simulink model "Allapotvisszacsatolas"  (Simulink 8.7)
settings: Solver=VariableStepAuto  StartTime=0.0  StopTime=T_sim  FixedStep=0.001  RelTol=1e-3
values from neighbouring files (symbols this model uses):
  d = 0.065    [Allapotvisszacsatolas_sim.m]
  delta_0 = deg2rad(delta_0)    [Allapotvisszacsatolas_sim.m]
  fi_0 = pi*fi_0*(SERVO_BAL-SERVO_JOBB)/(360*fi_m)    (= 0)    [Allapotvisszacsatolas_sim.m]
  fi_m = deg2rad(fi_m)    [Allapotvisszacsatolas_sim.m]
  k_delta = (L+d)/(kszi^2*d_5s^2)*(9*(L+d)-6*kszi^2*d_5s)    (= -0.808096379979)    [Allapotvisszacsatolas_sim.m]
  k_p = -9*(L+d)/(kszi^2*d_5s^2)    (= -3.12434564743)    [Allapotvisszacsatolas_sim.m]
  L = 0.22    [Allapotvisszacsatolas_sim.m]
  L_sensor = 0.13    [Allapotvisszacsatolas_sim.m]
  m = deg2rad(m)    [Allapotvisszacsatolas_sim.m]
  p_0 = 0.06    [Allapotvisszacsatolas_sim.m]
  p_1s = 0.0917605    [Allapotvisszacsatolas_sim.m]
  p_1TCRTa = 100    [Allapotvisszacsatolas_sim.m]
  p_1TCRTb = 3200    [Allapotvisszacsatolas_sim.m]
  p_2s = 0.068075    [Allapotvisszacsatolas_sim.m]
  p_2TCRTa = 100    [Allapotvisszacsatolas_sim.m]
  p_2TCRTb = 2400    [Allapotvisszacsatolas_sim.m]
  p_a = 0    [Allapotvisszacsatolas_sim.m]
  s_s = deg2rad(s_s)    [Allapotvisszacsatolas_sim.m]
  SERVO_BAL = 7250    [Allapotvisszacsatolas_sim.m]
  SERVO_JOBB = 4610    [Allapotvisszacsatolas_sim.m]
  T_delta = 0.003    [Allapotvisszacsatolas_sim.m]
  T_H = 0.03    [Allapotvisszacsatolas_sim.m]
  T_M = 0.01    [Allapotvisszacsatolas_sim.m]
  T_p = 0.003    [Allapotvisszacsatolas_sim.m]
  T_PWM = 0.003    [Allapotvisszacsatolas_sim.m]
  v = 1.75    [Allapotvisszacsatolas_sim.m]
settings Model: Creator=Mester Ádám  LastModifiedBy=Mester Ádám
settings DataIOCC: LimitDataPoints=off  SaveFormat=Dataset
settings DebuggingCC: UnderspecifiedInitializationDetection=Simplified  MergeDetectMultiDrivingBlocksExec=error
settings HardwareCC: ProdBitPerPointer=64  ProdLargestAtomicFloat=Float  ProdIntDivRoundTo=Zero  ProdEndianess=LittleEndian  ProdWordSize=64  ProdHWDeviceType=Intel->x86-64 (Windows64)
settings ModelReferenceCC: PropagateSignalLabelsOutOfModel=on
settings ConfigComp: CovModelRefEnable=off

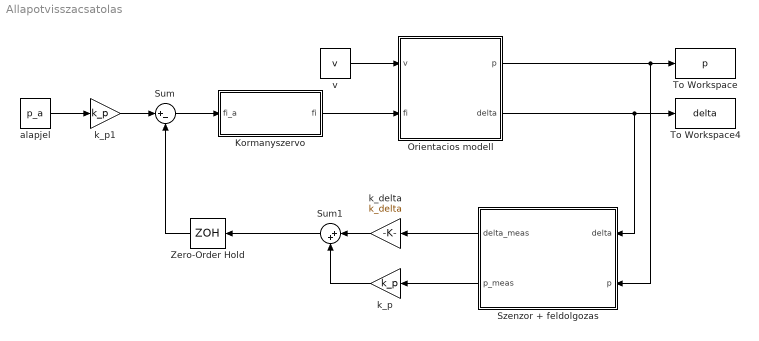
== system Allapotvisszacsatolas ==
  Kormanyszervo : Subsystem
  Orientacios modell : Subsystem
  Sum : Sum  Inputs=|+-
  Sum1 : Sum  Inputs=|++
  Szenzor + feldolgozas : Subsystem
  To Workspace : ToWorkspace  VariableName=p  SaveFormat=Structure With Time  SampleTime=-1
  To Workspace4 : ToWorkspace  VariableName=delta  SaveFormat=Structure With Time  SampleTime=-1
  Zero-Order Hold : ZeroOrderHold  SampleTime=T_PWM
  alapjel : Constant  Value=p_a
  k_delta : Gain  Gain=k_delta
  k_p : Gain  Gain=k_p
  k_p1 : Gain  Gain=k_p
  v : Constant  Value=v
  wires:
  Sum/1 -> Kormanyszervo/1(fi_a)
  v/1 -> Orientacios modell/1(v)
  k_delta/1 -> Sum1/1
  k_p/1 -> Sum1/2
  Szenzor + feldolgozas/2(p_meas) -> k_p/1
  Szenzor + feldolgozas/1(delta_meas) -> k_delta/1
  Orientacios modell/2(delta) -> To Workspace4/1, Szenzor + feldolgozas/1(delta)
  Orientacios modell/1(p) -> To Workspace/1, Szenzor + feldolgozas/2(p)
  k_p1/1 -> Sum/1
  Sum1/1 -> Zero-Order Hold/1
  Zero-Order Hold/1 -> Sum/2
  Kormanyszervo/1(fi) -> Orientacios modell/2(fi)
  alapjel/1 -> k_p1/1

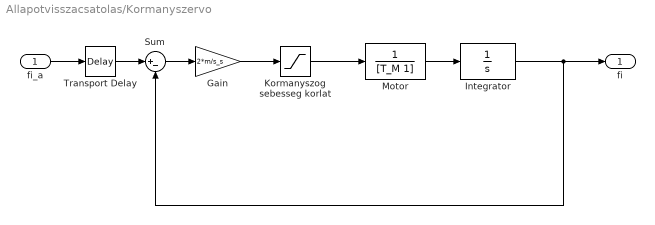
== system Allapotvisszacsatolas/Kormanyszervo ==
  fi_a : Inport
  Gain : Gain  Gain=2*m/s_s
  Integrator : Integrator  InitialCondition=fi_0
  Kormanyszog sebesseg korlat : Saturate  UpperLimit=abs(SERVO_BAL-SERVO_JOBB)*m/(2*fi_m)  LowerLimit=-abs(SERVO_BAL-SERVO_JOBB)*m/(2*fi_m)
  Motor : TransferFcn  Denominator=[T_M 1]
  Sum : Sum  Inputs=|+-
  Transport Delay : TransportDelay  DelayTime=T_H
  fi : Outport
  wires:
  fi_a/1 -> Transport Delay/1
  Transport Delay/1 -> Sum/1
  Sum/1 -> Gain/1
  Gain/1 -> Kormanyszog sebesseg korlat/1
  Kormanyszog sebesseg korlat/1 -> Motor/1
  Motor/1 -> Integrator/1
  Integrator/1 -> Sum/2, fi/1

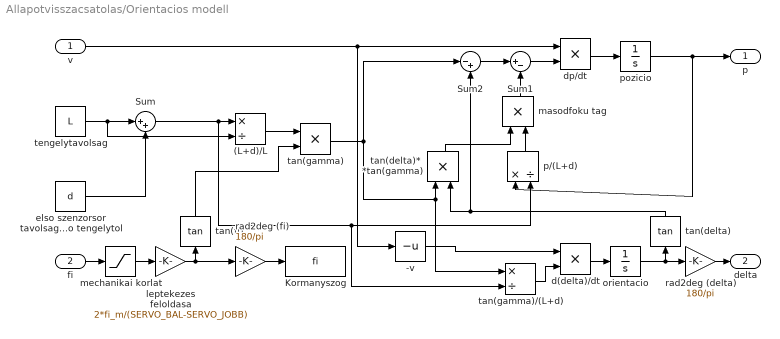
== system Allapotvisszacsatolas/Orientacios modell ==
  v : Inport
  fi : Inport  Port=2
  (L+d)/L : Product  Inputs=*/
  -v : UnaryMinus
  Kormanyszog : ToWorkspace  VariableName=fi  SaveFormat=Structure With Time  SampleTime=-1
  Sum : Sum  Inputs=|++
  Sum1 : Sum  Inputs=|+-
  Sum2 : Sum  Inputs=|-+
  d(delta)/dt : Product
  dp/dt : Product
  elso szenzorsor tavolsaga az elso tengelytol : Constant  Value=d
  leptekezes feloldasa : Gain  Gain=2*fi_m/(SERVO_BAL-SERVO_JOBB)
  masodfoku tag : Product
  mechanikai korlat : Saturate  UpperLimit=max(SERVO_JOBB,SERVO_BAL)-(SERVO_JOBB+SERVO_BAL)/2  LowerLimit=min(SERVO_JOBB,SERVO_BAL)-(SERVO_JOBB+SERVO_BAL)/2
  orientacio : Integrator  InitialCondition=delta_0
  p/(L+d) : Product  Inputs=*/
  pozicio : Integrator  InitialCondition=p_0
  rad2deg (delta) : Gain  Gain=180/pi
  rad2deg (fi) : Gain  Gain=180/pi
  tan(delta) : Trigonometry  Operator=tan
  tan(delta)*  *tan(gamma) : Product
  tan(fi) : Trigonometry  Operator=tan
  tan(gamma) : Product
  tan(gamma)/(L+d) : Product  Inputs=*/
  tengelytavolsag : Constant  Value=L
  p : Outport
  delta : Outport  Port=2
  wires:
  pozicio/1 -> p/1, p/(L+d)/1
  orientacio/1 -> rad2deg (delta)/1, tan(delta)/1
  dp/dt/1 -> pozicio/1
  v/1 -> -v/1, dp/dt/1
  tengelytavolsag/1 -> (L+d)/L/2, Sum/1
  elso szenzorsor tavolsaga az elso tengelytol/1 -> Sum/2
  Sum/1 -> (L+d)/L/1, p/(L+d)/2, tan(gamma)/(L+d)/2
  Sum1/1 -> dp/dt/2
  Sum2/1 -> Sum1/1
  tan(delta)/1 -> tan(delta)*  *tan(gamma)/2, Sum2/2
  masodfoku tag/1 -> Sum1/2
  p/(L+d)/1 -> masodfoku tag/2
  tan(delta)*  *tan(gamma)/1 -> masodfoku tag/1
  d(delta)/dt/1 -> orientacio/1
  tan(gamma)/(L+d)/1 -> d(delta)/dt/2
  -v/1 -> d(delta)/dt/1
  rad2deg (fi)/1 -> Kormanyszog/1
  (L+d)/L/1 -> tan(gamma)/1
  tan(fi)/1 -> tan(gamma)/2
  rad2deg (delta)/1 -> delta/1
  tan(gamma)/1 -> tan(delta)*  *tan(gamma)/1, tan(gamma)/(L+d)/1, Sum2/1
  leptekezes feloldasa/1 -> tan(fi)/1, rad2deg (fi)/1
  fi/1 -> mechanikai korlat/1
  mechanikai korlat/1 -> leptekezes feloldasa/1

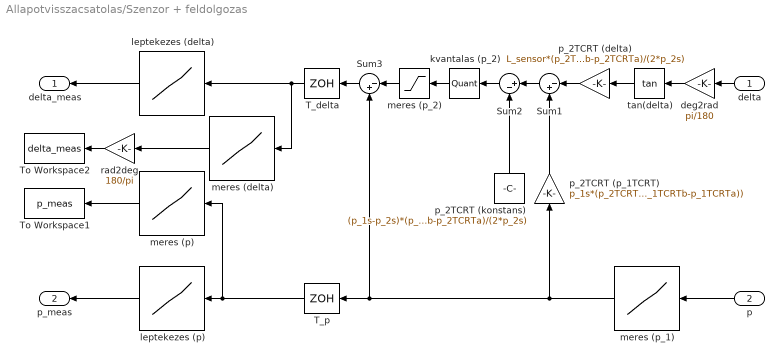
== system Allapotvisszacsatolas/Szenzor + feldolgozas ==
  delta : Inport
  p : Inport  Port=2
  Sum1 : Sum  Inputs=|-+
  Sum2 : Sum  Inputs=|+-
  Sum3 : Sum  Inputs=|-+
  T_delta : ZeroOrderHold  SampleTime=T_delta
  T_p : ZeroOrderHold  SampleTime=T_p
  To Workspace1 : ToWorkspace  VariableName=p_meas  SaveFormat=Structure With Time  SampleTime=-1
  To Workspace2 : ToWorkspace  VariableName=delta_meas  SaveFormat=Structure With Time  SampleTime=-1
  deg2rad : Gain  Gain=pi/180
  kvantalas (p_2) : Quantizer  QuantizationInterval=1
  leptekezes (delta) : Lookup_n-D  NumberOfTableDimensions=1  BreakpointsForDimension1=[min(p_1TCRTa-p_2TCRTb,p_1TCRTb-p_2TCRTa):max(p_1TCRTa-p_2TCRTb,p_1TCRTb-p_2TCRTa)]  Table=L*(SERVO_BAL-SERVO_JOBB)*atan((2*p_1s*[min(p_1TCRTa-p_2TCRTb,p_1TCRTb-p_2TCRTa):max(p_1TCRTa-p_2TCRTb,p_1TCRTb-p_2TCRTa)]/(p_1TCRTb-p_1TCRTa)-p_1s*(p_1TCRTb+p_1TCRTa)/(p_1TCRTb-p_1TCRTa)+p_2s*(p_2TCRTb+p_2TCRTa)/(p_2TCRTb-p_2TCRTa))/L_sensor)/(2*fi_m*(L+d))  InterpMethod=Nearest  InternalRulePriority=Speed  RndMeth=Simplest  InputSameDT=on
  leptekezes (p) : Lookup_n-D  NumberOfTableDimensions=1  BreakpointsForDimension1=[min(p_1TCRTa,p_1TCRTb):max(p_1TCRTa,p_1TCRTb)]  Table=L*(SERVO_BAL-SERVO_JOBB)*p_1s*(2*[min(p_1TCRTa,p_1TCRTb):max(p_1TCRTa,p_1TCRTb)]-p_1TCRTb-p_1TCRTa)/(2*fi_m*(L+d)*(p_1TCRTb-p_1TCRTa))  InterpMethod=Nearest  InternalRulePriority=Speed  RndMeth=Simplest  InputSameDT=on
  meres (delta) : Lookup_n-D  NumberOfTableDimensions=1  BreakpointsForDimension1=[min(p_1TCRTa-p_2TCRTb,p_1TCRTb-p_2TCRTa):max(p_1TCRTa-p_2TCRTb,p_1TCRTb-p_2TCRTa)]  Table=atan((2*p_1s*[min(p_1TCRTa-p_2TCRTb,p_1TCRTb-p_2TCRTa):max(p_1TCRTa-p_2TCRTb,p_1TCRTb-p_2TCRTa)]/(p_1TCRTb-p_1TCRTa)-p_1s*(p_1TCRTb+p_1TCRTa)/(p_1TCRTb-p_1TCRTa)+p_2s*(p_2TCRTb+p_2TCRTa)/(p_2TCRTb-p_2TCRTa))/L_sensor)  InterpMethod=Nearest  InternalRulePriority=Speed  RndMeth=Simplest  InputSameDT=on
  meres (p) : Lookup_n-D  NumberOfTableDimensions=1  BreakpointsForDimension1=[min(p_1TCRTa,p_1TCRTb):max(p_1TCRTa,p_1TCRTb)]  Table=p_1s*(2*[min(p_1TCRTa,p_1TCRTb):max(p_1TCRTa,p_1TCRTb)]-p_1TCRTb-p_1TCRTa)/(p_1TCRTb-p_1TCRTa)  InterpMethod=Nearest  InternalRulePriority=Speed  RndMeth=Simplest  InputSameDT=on
  meres (p_1) : Lookup_n-D  NumberOfTableDimensions=1  BreakpointsForDimension1=[-p_1s:2*p_1s/abs(p_1TCRTb-p_1TCRTa):p_1s]  Table=round([-p_1s:2*p_1s/abs(p_1TCRTb-p_1TCRTa):p_1s]*(p_1TCRTb-p_1TCRTa)/(2*p_1s)+(p_1TCRTb+p_1TCRTa)/2)  InterpMethod=Nearest  InternalRulePriority=Speed  RndMeth=Simplest  InputSameDT=on
  meres (p_2) : Saturate  UpperLimit=max(p_2TCRTa,p_2TCRTb)  LowerLimit=min(p_2TCRTa,p_2TCRTb)
  p_2TCRT (delta) : Gain  Gain=L_sensor*(p_2TCRTb-p_2TCRTa)/(2*p_2s)
  p_2TCRT (konstans) : Constant  Value=(p_1s-p_2s)*(p_2TCRTb-p_2TCRTa)/(2*p_2s)
  p_2TCRT (p_1TCRT) : Gain  Gain=p_1s*(p_2TCRTb-p_2TCRTa)/(p_2s*(p_1TCRTb-p_1TCRTa))
  rad2deg : Gain  Gain=180/pi
  tan(delta) : Trigonometry  Operator=tan
  delta_meas : Outport
  p_meas : Outport  Port=2
  wires:
  leptekezes (p)/1 -> p_meas/1
  leptekezes (delta)/1 -> delta_meas/1
  p/1 -> meres (p_1)/1
  meres (p_1)/1 -> T_p/1, Sum3/2, p_2TCRT (p_1TCRT)/1
  delta/1 -> deg2rad/1
  deg2rad/1 -> tan(delta)/1
  tan(delta)/1 -> p_2TCRT (delta)/1
  Sum1/1 -> Sum2/1
  p_2TCRT (konstans)/1 -> Sum2/2
  p_2TCRT (delta)/1 -> Sum1/1
  p_2TCRT (p_1TCRT)/1 -> Sum1/2
  Sum2/1 -> kvantalas (p_2)/1
  meres (p)/1 -> To Workspace1/1
  rad2deg/1 -> To Workspace2/1
  meres (delta)/1 -> rad2deg/1
  T_p/1 -> leptekezes (p)/1, meres (p)/1
  Sum3/1 -> T_delta/1
  T_delta/1 -> leptekezes (delta)/1, meres (delta)/1
  meres (p_2)/1 -> Sum3/1
  kvantalas (p_2)/1 -> meres (p_2)/1
